simulink model "second_order"  (R2023b)
settings: Solver=VariableStepAuto  StartTime=0.0  StopTime=10.0  RelTol=1e-3
settings Model: Creator=ascom  LastModifiedBy=ascom

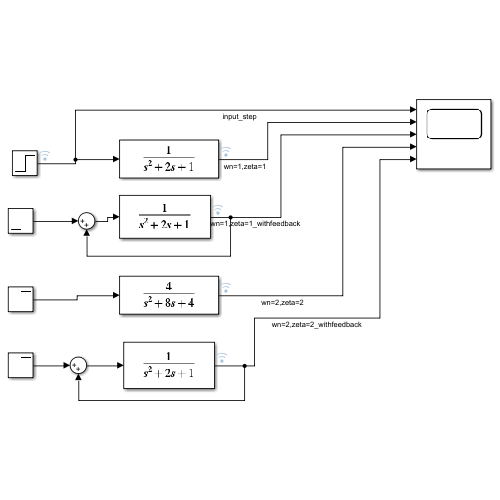
[thumbnail: Simulink's stored preview of the top-level diagram]
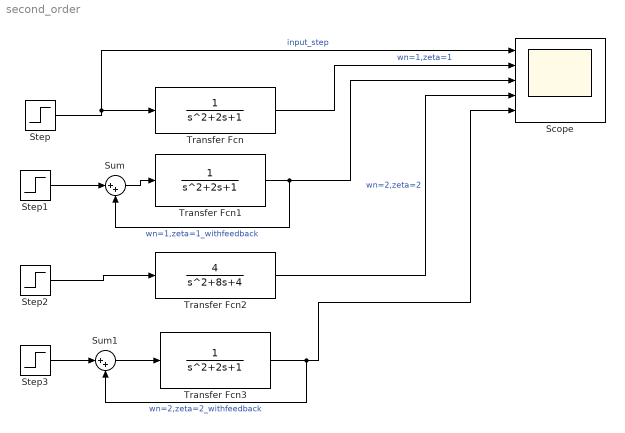
== system second_order ==
  Scope : Scope  NumInputPorts=5
  Step{,1..3} (4 alike) : Step  SampleTime=0
  Sum : Sum  Inputs=|++
  Sum1 : Sum  Inputs=|++
  Transfer Fcn : TransferFcn
  Transfer Fcn1 : TransferFcn
  Transfer Fcn2 : TransferFcn  Numerator=[4]  Denominator=[1 8 4]
  Transfer Fcn3 : TransferFcn
  wires:
  Step/1 -> Scope/1, Transfer Fcn/1  "input_step"
  Transfer Fcn/1 -> Scope/2  "wn=1,zeta=1"
  Sum/1 -> Transfer Fcn1/1
  Step1/1 -> Sum/1
  Transfer Fcn1/1 -> Sum/2, Scope/3  "wn=1,zeta=1_withfeedback"
  Step2/1 -> Transfer Fcn2/1
  Transfer Fcn2/1 -> Scope/4  "wn=2,zeta=2"
  Step3/1 -> Sum1/1
  Sum1/1 -> Transfer Fcn3/1
  Transfer Fcn3/1 -> Sum1/2, Scope/5  "wn=2,zeta=2_withfeedback"
